simulink model "three_NSMC"  (R2021b)
settings: Solver=ode8  StartTime=0.0  StopTime=10  FixedStep=10^(-4)  MaxStep=10-4  RelTol=1e-3
settings Model: Creator=wkw  LastModifiedBy=wkw

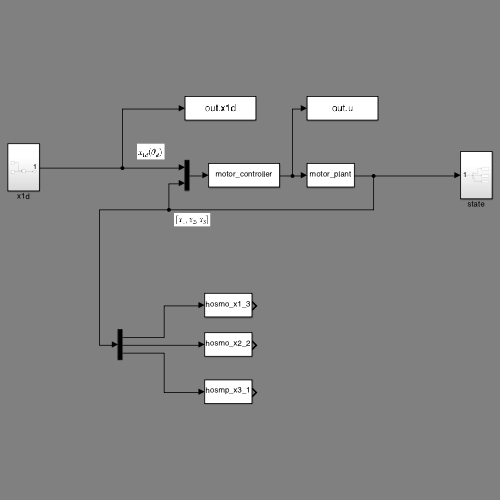
[thumbnail: Simulink's stored preview of the top-level diagram]
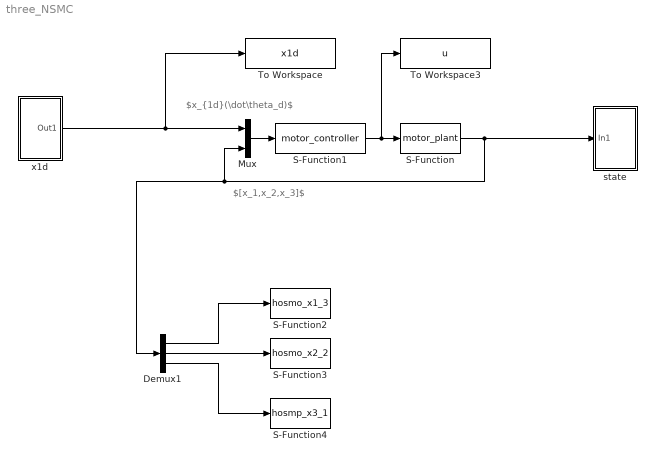
== system three_NSMC ==
  note: $[x_1,x_2,x_3]$
  note: $x_{1d}(\dot\theta_d)$
  Demux1 : Demux  Outputs=3
  Mux : Mux  Inputs=2
  S-Function : S-Function  FunctionName=motor_plant  SFunctionDeploymentMode=off  EnableBusSupport=off
  S-Function1 : S-Function  FunctionName=motor_controller  SFunctionDeploymentMode=off  EnableBusSupport=off
  S-Function2 : S-Function  FunctionName=hosmo_x1_3  SFunctionDeploymentMode=off  EnableBusSupport=off
  S-Function3 : S-Function  FunctionName=hosmo_x2_2  SFunctionDeploymentMode=off  EnableBusSupport=off
  S-Function4 : S-Function  FunctionName=hosmp_x3_1  SFunctionDeploymentMode=off  EnableBusSupport=off
  To Workspace : ToWorkspace  VariableName=x1d  SaveFormat=Timeseries  SampleTime=-1
  To Workspace3 : ToWorkspace  VariableName=u  SaveFormat=Timeseries  SampleTime=-1
  state : Subsystem
  x1d : Subsystem
  wires:
  Mux/1 -> S-Function1/1
  S-Function/1 -> state/1(In1), Demux1/1, Mux/2
  S-Function1/1 -> To Workspace3/1, S-Function/1
  Demux1/1 -> S-Function2/1
  Demux1/2 -> S-Function3/1
  Demux1/3 -> S-Function4/1
  x1d/1(Out1) -> To Workspace/1, Mux/1

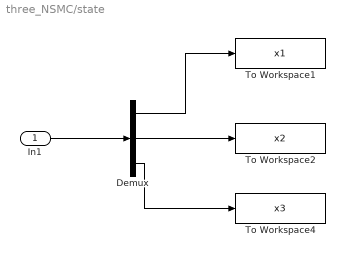
== system three_NSMC/state ==
  In1 : Inport
  Demux : Demux  Outputs=3
  To Workspace1 : ToWorkspace  VariableName=x1  SaveFormat=Timeseries  SampleTime=-1
  To Workspace2 : ToWorkspace  VariableName=x2  SaveFormat=Timeseries  SampleTime=-1
  To Workspace4 : ToWorkspace  VariableName=x3  SaveFormat=Timeseries  SampleTime=-1
  wires:
  In1/1 -> Demux/1
  Demux/3 -> To Workspace4/1
  Demux/1 -> To Workspace1/1
  Demux/2 -> To Workspace2/1

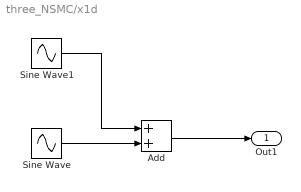
== system three_NSMC/x1d ==
  Add : Sum
  Sine Wave : Sin  Amplitude=0.5  SampleTime=0
  Sine Wave1 : Sin  Amplitude=0.5  Frequency=0.5  SampleTime=0
  Out1 : Outport
  wires:
  Add/1 -> Out1/1
  Sine Wave/1 -> Add/2
  Sine Wave1/1 -> Add/1
